simulink model "Dynamics"  (R2024b)
settings: Solver=VariableStepAuto  StartTime=0.0  StopTime=30  RelTol=1e-3
undefined symbols (not defined in the file): bball_mass, SimInDyn
libraries: simulink x2, matrix_library x1
settings Model: Creator=macheson  LastModifiedBy=macheson

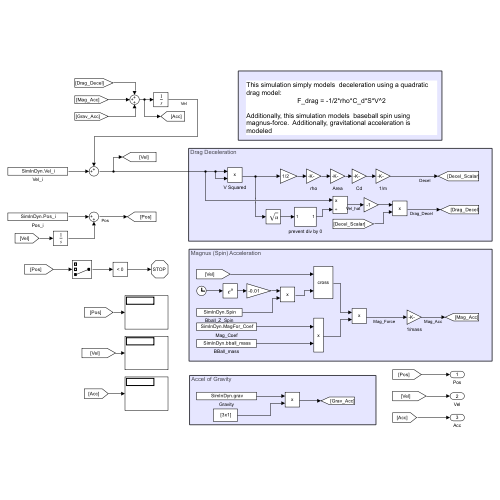
[thumbnail: Simulink's stored preview of the top-level diagram]
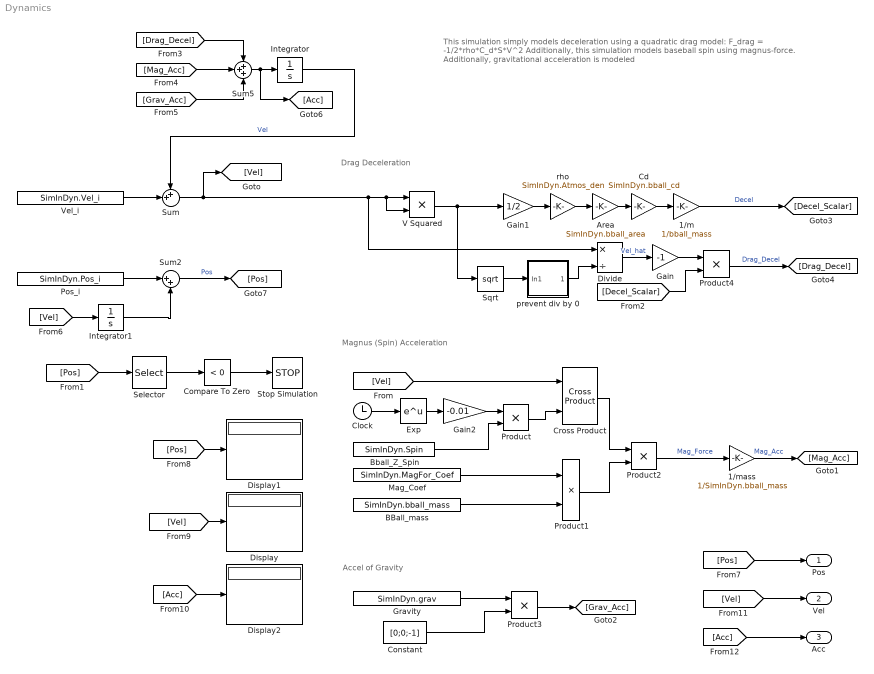
== system Dynamics ==
  note: Accel of Gravity
  note: Magnus (Spin) Acceleration
  note: This simulation simply models deceleration using a quadratic drag model:
      | F_drag = -1/2*rho*C_d*S*V^2
      |
      | Additionally, this simulation models baseball spin using magnus-force. Additionally, gravitational acceleration is modeled
  note: Drag Deceleration
  1/m : Gain  Gain=1/bball_mass
  1/mass : Gain  Gain=1/SimInDyn.bball_mass
  Area : Gain  Gain=SimInDyn.bball_area
  BBall_mass : Constant  Value=SimInDyn.bball_mass
  Bball_Z_Spin : Constant  Value=SimInDyn.Spin
  Cd : Gain  Gain=SimInDyn.bball_cd
  Clock : Clock
  Compare To Zero : simulink/Logic and Bit Operations/Compare To Zero  relop=<  OutDataTypeStr=boolean
  Constant : Constant  Value=[0;0;-1]
  Cross Product : matrix_library/Cross Product
  Display : Display
  Display1 : Display
  Display2 : Display
  Divide : Product  Inputs=*/
  Exp : Math
  Gain : Gain  Gain=-1
  Gain1 : Gain  Gain=1/2
  Gain2 : Gain  Gain=-0.01
  Gravity : Constant  Value=SimInDyn.grav
  Integrator : Integrator
  Integrator1 : Integrator
  Mag_Coef : Constant  Value=SimInDyn.MagFor_Coef
  Pos_i : Constant  Value=SimInDyn.Pos_i
  Product{,1..4} (5 alike) : Product
  Selector : Selector  InputPortWidth=3  IndexOptions=Index vector (dialog)  Indices=[3]  OutputSizes=1
  Sqrt : Sqrt
  Stop Simulation : Stop
  Sum : Sum  Inputs=++|
  Sum2 : Sum  Inputs=|++
  Sum5 : Sum  Inputs=+++
  V Squared : Product
  Vel_i : Constant  Value=SimInDyn.Vel_i
  prevent div by 0 : Subsystem
  rho : Gain  Gain=SimInDyn.Atmos_den
  Pos : Outport
  Vel : Outport  Port=2
  Acc : Outport  Port=3
  wires:
  Integrator/1 -> Sum/1  "Vel"
  Vel_i/1 -> Sum/2
  Cd/1 -> 1/m/1
  V Squared/1 -> Sqrt/1, Gain1/1
  Integrator1/1 -> Sum2/2
  Gain1/1 -> rho/1
  rho/1 -> Area/1
  1/m/1 -> [Decel_Scalar]  "Decel"
  Area/1 -> Cd/1
  Sum/1 -> V Squared/1, V Squared/2, Divide/1, [Vel]
  Bball_Z_Spin/1 -> Product/2
  [Vel] -> Cross Product/1
  Mag_Coef/1 -> Product1/1
  BBall_mass/1 -> Product1/2
  Cross Product/1 -> Product2/1
  Product1/1 -> Product2/2
  Product2/1 -> 1/mass/1  "Mag_Force"
  1/mass/1 -> [Mag_Acc]  "Mag_Acc"
  Gravity/1 -> Product3/1
  Constant/1 -> Product3/2
  Product3/1 -> [Grav_Acc]
  Divide/1 -> Gain/1  "Vel_hat"
  Gain/1 -> Product4/1
  [Decel_Scalar] -> Product4/2
  Product4/1 -> [Drag_Decel]  "Drag_Decel"
  Sum5/1 -> [Acc], Integrator/1
  [Drag_Decel] -> Sum5/1
  [Mag_Acc] -> Sum5/2
  [Grav_Acc] -> Sum5/3
  [Vel] -> Integrator1/1
  Pos_i/1 -> Sum2/1
  Sum2/1 -> [Pos]  "Pos"
  [Pos] -> Pos/1
  [Pos] -> Display1/1
  [Vel] -> Display/1
  [Acc] -> Display2/1
  [Vel] -> Vel/1
  [Acc] -> Acc/1
  Sqrt/1 -> prevent div by 0/1(In1)
  prevent div by 0/1(Out1) -> Divide/2
  [Pos] -> Selector/1
  Selector/1 -> Compare To Zero/1
  Compare To Zero/1 -> Stop Simulation/1
  Exp/1 -> Gain2/1
  Clock/1 -> Exp/1
  Gain2/1 -> Product/1
  Product/1 -> Cross Product/2

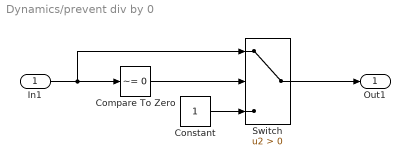
== system Dynamics/prevent div by 0 ==
  In1 : Inport
  Compare To Zero : simulink/Logic and Bit Operations/Compare To Zero  relop=~=  OutDataTypeStr=boolean
  Constant : Constant
  Switch : Switch  Criteria=u2 > Threshold  SaturateOnIntegerOverflow=off  InputSameDT=off
  Out1 : Outport  VectorParamsAs1DForOutWhenUnconnected=off
  wires:
  In1/1 -> Compare To Zero/1, Switch/1
  Compare To Zero/1 -> Switch/2
  Constant/1 -> Switch/3
  Switch/1 -> Out1/1
